simulink model "solve_para"  (Simulink 6.0)
settings: Solver=FixedStepDiscrete  SolverMode=SingleTasking  StartTime=0.0  StopTime=0.0001  RelTol=1e-3  AbsTol=1e-6
undefined symbols (not defined in the file or in its folder): a0, alpha0, b0, c0, e0, HT
settings Model: Creator=silvano  LastModifiedBy=batserve  ExtModeTrigMode=oneshot  ExtModeArmWhenConnect=off  ExtModeAutoUpdateStatusClock=off
settings DataIOCC: FinalStateName=XF  LimitDataPoints=off  TimeSaveName=t  SignalLoggingName=sigsOut
settings OptimizationCC: BlockReduction=off  BooleanDataType=off
settings DebuggingCC: AlgebraicLoopMsg=none  SolverPrmCheckMsg=none
settings HardwareCC: TargetUnknown=on
settings RTWCC: TemplateMakefile=grt_vc.tmf

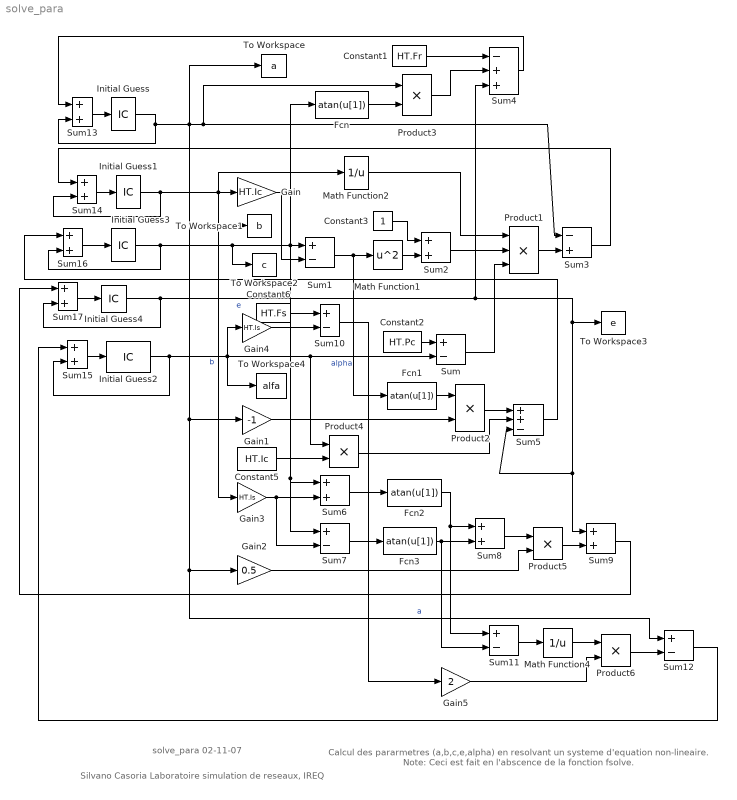
== system solve_para ==
  note: Silvano Casoria
      | Laboratoire simulation de reseaux, IREQ
  note: solve_para
      | 02-11-07
  note: Calcul des pararmetres (a,b,c,e,alpha) en resolvant un systeme d'equation non-lineaire.
      | Note: Ceci est fait en l'abscence de la fonction fsolve.
  Constant1 : Constant  Value=HT.Fr
  Constant2 : Constant  Value=HT.Pc
  Constant3 : Constant
  Constant5 : Constant  Value=HT.Ic
  Constant6 : Constant  Value=HT.Fs
  Fcn{,1..3} (4 alike) : Fcn  Expr=atan(u[1])
  Gain : Gain  Gain=HT.Ic  SaturateOnIntegerOverflow=on
  Gain1 : Gain  Gain=-1  SaturateOnIntegerOverflow=on
  Gain2 : Gain  Gain=0.5  SaturateOnIntegerOverflow=on
  Gain3 : Gain  Gain=HT.Is  SaturateOnIntegerOverflow=on
  Gain4 : Gain  Gain=HT.Is  SaturateOnIntegerOverflow=on
  Gain5 : Gain  Gain=2  SaturateOnIntegerOverflow=on
  Initial Guess : InitialCondition  Value=a0
  Initial Guess1 : InitialCondition  Value=b0
  Initial Guess2 : InitialCondition  Value=alpha0
  Initial Guess3 : InitialCondition  Value=c0
  Initial Guess4 : InitialCondition  Value=e0
  Math Function1 : Math  Operator=square  SaturateOnIntegerOverflow=on
  Math Function2 : Math  Operator=reciprocal  SaturateOnIntegerOverflow=on
  Math Function4 : Math  Operator=reciprocal  SaturateOnIntegerOverflow=on
  Product1 : Product  Inputs=3  SaturateOnIntegerOverflow=on  InputSameDT=on
  Product{2..6} (5 alike) : Product  SaturateOnIntegerOverflow=on  InputSameDT=on
  Sum{,1,7,10..12} (6 alike) : Sum  Inputs=+-  SaturateOnIntegerOverflow=on  InputSameDT=on
  Sum{2,6,8..9,13..17} (9 alike) : Sum  SaturateOnIntegerOverflow=on  InputSameDT=on
  Sum3 : Sum  Inputs=-+  SaturateOnIntegerOverflow=on  InputSameDT=on
  Sum4 : Sum  Inputs=-++  SaturateOnIntegerOverflow=on  InputSameDT=on
  Sum5 : Sum  Inputs=++-  SaturateOnIntegerOverflow=on  InputSameDT=on
  To Workspace : ToWorkspace  VariableName=a  SampleTime=-1  SaveFormat=Array
  To Workspace1 : ToWorkspace  VariableName=b  SampleTime=-1  SaveFormat=Array
  To Workspace2 : ToWorkspace  VariableName=c  SampleTime=-1  SaveFormat=Array
  To Workspace3 : ToWorkspace  VariableName=e  SampleTime=-1  SaveFormat=Array
  To Workspace4 : ToWorkspace  VariableName=alfa  SampleTime=-1  SaveFormat=Array
  wires:
  Initial Guess2/1 -> Sum15/2, Sum/2, Product4/1, Gain4/1, To Workspace4/1  "alpha"
  Sum15/1 -> Initial Guess2/1
  Initial Guess4/1 -> Sum17/2, Sum4/3, To Workspace3/1, Sum9/1, Sum5/3  "e"
  Sum17/1 -> Initial Guess4/1
  Initial Guess3/1 -> Sum16/2, Fcn/1, Sum1/1, Sum6/1, Sum7/1, To Workspace2/1
  Sum16/1 -> Initial Guess3/1
  Initial Guess1/1 -> Sum14/2, Gain/1, Math Function2/1, Gain3/1, To Workspace1/1  "b"
  Sum14/1 -> Initial Guess1/1
  Sum3/1 -> Sum14/1
  Initial Guess/1 -> Sum3/1, Product3/1, Gain1/1, Gain2/1, Sum12/1, To Workspace/1, Sum13/2  "a"
  Sum13/1 -> Initial Guess/1
  Sum4/1 -> Sum13/1
  Gain/1 -> Sum1/2
  Math Function2/1 -> Product1/1
  Sum2/1 -> Product1/2
  Fcn/1 -> Product3/2
  Constant1/1 -> Sum4/1
  Product3/1 -> Sum4/2
  Constant2/1 -> Sum/1
  Sum/1 -> Product1/3
  Product1/1 -> Sum3/2
  Sum1/1 -> Math Function1/1, Fcn1/1
  Fcn1/1 -> Product2/1
  Gain1/1 -> Product2/2
  Constant5/1 -> Product4/2
  Product2/1 -> Sum5/1
  Product4/1 -> Sum5/2
  Sum5/1 -> Sum16/1
  Sum6/1 -> Fcn2/1
  Gain3/1 -> Sum6/2, Sum7/2
  Sum7/1 -> Fcn3/1
  Sum8/1 -> Product5/1
  Gain2/1 -> Product5/2
  Product5/1 -> Sum9/2
  Sum9/1 -> Sum17/1
  Gain4/1 -> Sum10/2
  Constant6/1 -> Sum10/1
  Math Function1/1 -> Sum2/2
  Constant3/1 -> Sum2/1
  Fcn2/1 -> Sum8/1, Sum11/1
  Fcn3/1 -> Sum8/2, Sum11/2
  Sum11/1 -> Math Function4/1
  Sum10/1 -> Gain5/1
  Math Function4/1 -> Product6/1
  Gain5/1 -> Product6/2
  Product6/1 -> Sum12/2
  Sum12/1 -> Sum15/1
